simulink model "Main_ekart"  (R2021b)
settings: Solver=FixedStepAuto  StartTime=0.0  StopTime=inf  FixedStep=1/500  RelTol=1e-3  EnableMultiTasking=on
values from neighbouring files (symbols this model uses):
  a = [1 -2.62355180661 2.31468258109 -0.685535977285]    [IMU_filt_100Hz.mat]    (also in IMU_filt_500Hz.mat = [1 -2.92460623545 2.85202781859 -0.92736996835])
  angles = [0 4.9 5 10 15 20 25 30 35 40]    [CreateAllControllers.m]
  b = [0.000699349649901 0.0020980489497 0.0020980489497 0.000699349649901]    [IMU_filt_100Hz.mat]    (also in IMU_filt_500Hz.mat = [6.45184912909e-06 1.93555473873e-05 1.93555473873e-05 6.451)
  D = (DMFx+DMFy)/2    (= 1.2194)    [kart_parameters2.m]
  gear_ratio = 3.2    [kart_parameters2.m]
  L = sys*C    [build_controller_PI.m]    (also in kart_parameters2.m = 1.042)
  newcurrent = [-186.423 -186.283922965 -186.14484593 -186.005768895 -185.866691861 -185.727614826 -185.588537791 -185.449460756 -185.310383721 -185.171306686 -185.032229652 -184.893152617 ... (1000 elements, 1x1000)]    [Torque_map.mat]
  newtorque = [-28.1755 -28.1190925926 -28.0626851852 -28.0062777778 -27.9498703704 -27.893462963 -27.8370555556 -27.7806481481 -27.7242407407 -27.6678333333 -27.6114259259 -27.5550185185 ... (1000 elements, 1x1000)]    [Torque_map.mat]
  percent = [0 0.1001001001 0.2002002002 0.3003003003 0.4004004004 0.500500500501 0.600600600601 0.700700700701 0.800800800801 0.900900900901 1.001001001 1.1011011011 ... (1000 elements, 1x1000)]    [Torque_accel.mat]
  speeds = [0 19.9 20 30 40]    [CreateAllControllers.m]
  table_i = [zeros(1,10) ... (first row only)    [CreateAllControllers.m]
  table_p = [zeros(1, 10) ... (first row only)    [CreateAllControllers.m]
  torque = [0.1025 0.130601101101 0.158702202202 0.186803303303 0.214904404404 0.243005505506 0.271106606607 0.299207707708 0.327308808809 0.35540990991 0.383511011011 0.411612112112 ... (1000 elements, 1x1000)]    [Torque_accel.mat]
libraries: simulink x50, mcp2515lib x46, etargetslib x4, svdutilitieslib x3, cstblocks x2, slpidlib x1
(part 1 of 4)
settings Model: Creator=s393429  LastModifiedBy=maximesabbadini
settings SolverCC: PositivePriorityOrder=on
settings OptimizationCC: EnhancedBackFolding=on  PassReuseOutputArgsThreshold=0  MaxStackSize=64  OptimizeBlockOrder=speed  DifferentSizesBufferReuse=on  OptimizationCustomize=off
settings DebuggingCC: ParameterTunabilityLossMsg=error  UnconnectedInputMsg=none  UnconnectedOutputMsg=none  UnconnectedLineMsg=none
settings HardwareCC: ProdBitPerPointer=32  ProdBitPerSizeT=32  ProdBitPerPtrDiffT=32  ProdLargestAtomicInteger=Long  ProdLargestAtomicFloat=Double  ProdWordSize=32  ProdLongLongMode=on  ProdHWDeviceType=ARM Compatible->ARM Cortex  UseEmbeddedCoderFeatures=off
settings RTWCC: Description=Embedded Coder  SystemTargetFile=ert.tlc  HardwareBoard=Raspberry Pi  TLCOptions="-aInlineSetEventsForThisBaseRateFcn=TLC_FALSE -aSuppressMultiTaskScheduler=TLC_FALSE  -aRateBasedStepFcn=0"  TemplateMakefile=ert_default_tmf  Toolchain=GNU GCC Embedded Linux  BuildConfiguration=Faster Runs  DLArmComputeVersion=20.02.1
settings CodeAppCC: ForceParamTrailComments=on  OperatorAnnotations=on
settings ERTTargetCC: ERTCustomFileBanners=off  SupportContinuousTime=on  SupportNonInlinedSFcns=on  RemoveResetFunc=off  SupportVariableSizeSignals=on  ModelStepFunctionPrototypeControlCompliant=off  ExtMode=on  ExtModeTransport=2  ExtModeStaticAlloc=on  ExtModeMexFile=ext_xcp  ExtModeMexArgs='192.168.8.1' 0 17725  ExtModeIntrfLevel=Level2 - Open  ERTSrcFileBannerTemplate=codertarget_code_template.cgt  ERTHdrFileBannerTemplate=codertarget_code_template.cgt  ERTDataSrcFileTemplate=codertarget_code_template.cgt  ERTDataHdrFileTemplate=codertarget_code_template.cgt

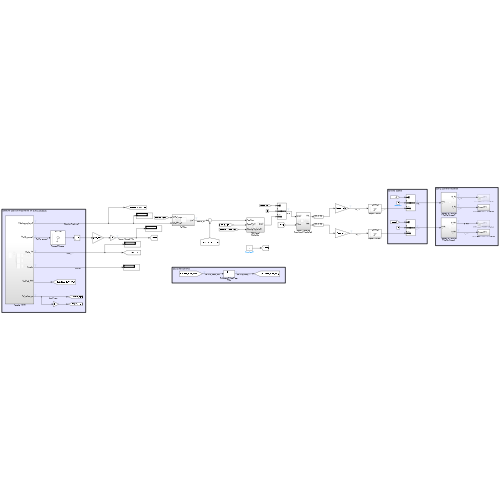
[thumbnail: Simulink's stored preview of the top-level diagram]
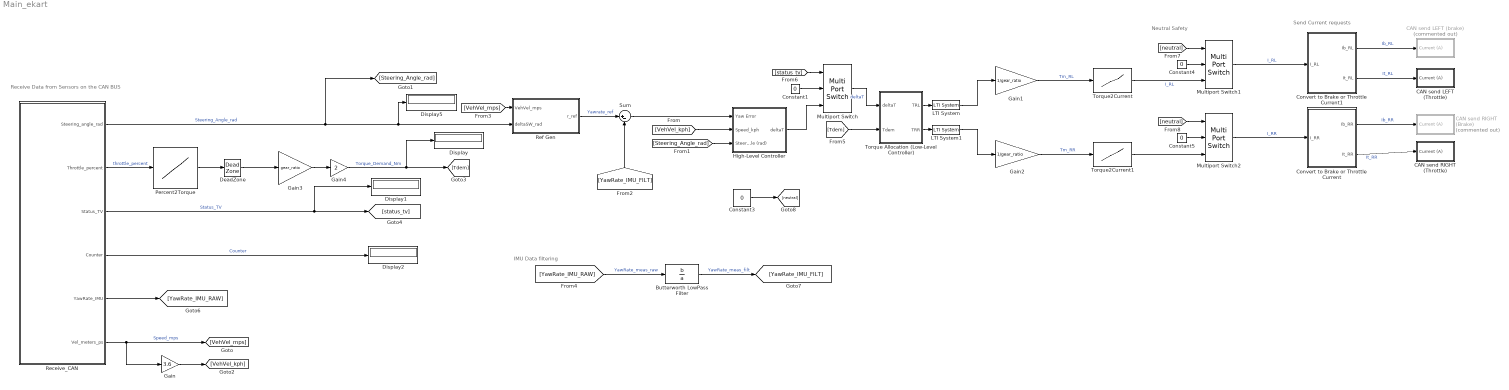
== system Main_ekart ==
  note: Send Current requests
  note: Neutral Safety
  note: IMU Data filtering
  note: Receive Data from Sensors on the CAN BUS
  Butterworth LowPass Filter : DiscreteTransferFcn  Numerator=b  Denominator=a
  CAN send LEFT (Throttle) : Subsystem
  CAN send LEFT (brake) : Subsystem  Commented=on
  CAN send RIGHT (Brake) : Subsystem  Commented=on
  CAN send RIGHT (Throttle) : Subsystem
  Constant1 : Constant  Value=0
  Constant3 : Constant  Value=0
  Constant4 : Constant  Value=0  OutDataTypeStr=int32
  Constant5 : Constant  Value=0  OutDataTypeStr=int32
  Convert to Brake or Throttle Current : Subsystem
  Convert to Brake or Throttle Current1 : Subsystem
  DeadZone : DeadZone  LowerValue=0  UpperValue=1  SaturateOnIntegerOverflow=on
  Display{,1..2,5} (4 alike) : Display
  Gain : Gain  Gain=3.6  OutDataTypeStr=Inherit: Inherit via back propagation
  Gain1 : Gain  Gain=1/gear_ratio
  Gain2 : Gain  Gain=1/gear_ratio
  Gain3 : Gain  Gain=gear_ratio
  Gain4 : Gain  Gain=2
  High-Level Controller : Subsystem
  LTI System : cstblocks/LTI System  sys=tf(5,[1 5])  IC=[]
  LTI System1 : cstblocks/LTI System  sys=tf(5,[1 5])  IC=[]
  Multiport Switch : MultiPortSwitch  DataPortOrder=Zero-based contiguous  Inputs=2  zeroidx=on
  Multiport Switch1 : MultiPortSwitch  DataPortOrder=Zero-based contiguous  Inputs=2  zeroidx=on
  Multiport Switch2 : MultiPortSwitch  DataPortOrder=Zero-based contiguous  Inputs=2  zeroidx=on
  Percent2Torque : Lookup_n-D  NumberOfTableDimensions=1  BreakpointsForDimension1=percent  Table=torque  InternalRulePriority=Speed  RndMeth=Simplest  InputSameDT=on
  Receive_CAN : Subsystem
  Ref Gen : Subsystem
  Sum : Sum  Inputs=|+-
  Torque Allocation (Low-Level Controller) : Subsystem
  Torque2Current : Lookup_n-D  NumberOfTableDimensions=1  BreakpointsForDimension1=newtorque  Table=newcurrent  InternalRulePriority=Speed  RndMeth=Simplest  InputSameDT=on
  Torque2Current1 : Lookup_n-D  NumberOfTableDimensions=1  BreakpointsForDimension1=newtorque  Table=newcurrent  InternalRulePriority=Speed  RndMeth=Simplest  InputSameDT=on
  wires:
  Constant1/1 -> Multiport Switch/2
  High-Level Controller/1(deltaT) -> Multiport Switch/3
  Sum/1 -> High-Level Controller/1(Yaw Error)
  Gain2/1 -> Torque2Current1/1  "Tm_RR"
  Gain1/1 -> Torque2Current/1  "Tm_RL"
  Ref Gen/1(r_ref) -> Sum/1  "Yawrate_ref"
  Torque Allocation (Low-Level Controller)/1(TRL) -> LTI System/1
  Torque Allocation (Low-Level Controller)/2(TRR) -> LTI System1/1
  Multiport Switch/1 -> Torque Allocation (Low-Level Controller)/1(deltaT)  "deltaT"
  [VehVel_kph] -> High-Level Controller/2(Speed_kph)
  [Steering_Angle_rad] -> High-Level Controller/3(Steering Angle (rad))
  [VehVel_mps] -> Ref Gen/1(VehVel_mps)
  Receive_CAN/4(Counter) -> Display2/1  "Counter"
  Percent2Torque/1 -> DeadZone/1
  Torque2Current1/1 -> Multiport Switch2/3
  [neutral] -> Multiport Switch2/1
  [neutral] -> Multiport Switch1/1
  Gain3/1 -> Gain4/1
  Gain4/1 -> [Tdem], Display/1  "Torque_Demand_Nm"
  Receive_CAN/1(Steering_angle_rad) -> [Steering_Angle_rad], Display5/1, Ref Gen/2(deltaSW_rad)  "Steering_Angle_rad"
  LTI System/1 -> Gain1/1
  LTI System1/1 -> Gain2/1
  Receive_CAN/3(Status_TV) -> [status_tv], Display1/1  "Status_TV"
  Convert to Brake or Throttle Current1/1(Ib_RL) -> CAN send LEFT (brake)/1(Current (A))  "Ib_RL"
  [Tdem] -> Torque Allocation (Low-Level Controller)/2(Tdem)
  Receive_CAN/6(Vel_meters_ps) -> Gain/1, [VehVel_mps]  "Speed_mps"
  Gain/1 -> [VehVel_kph]
  Receive_CAN/5(YawRate_IMU) -> [YawRate_IMU_RAW]
  [YawRate_IMU_FILT] -> Sum/2
  [status_tv] -> Multiport Switch/1
  [YawRate_IMU_RAW] -> Butterworth LowPass Filter/1  "YawRate_meas_raw"
  Butterworth LowPass Filter/1 -> [YawRate_IMU_FILT]  "YawRate_meas_filt"
  DeadZone/1 -> Gain3/1
  Convert to Brake or Throttle Current1/2(It_RL) -> CAN send LEFT (Throttle)/1(Current (A))  "It_RL"
  Constant3/1 -> [neutral]
  Convert to Brake or Throttle Current/2(It_RR) -> CAN send RIGHT (Throttle)/1(Current (A))  "It_RR"
  Receive_CAN/2(Throttle_percent) -> Percent2Torque/1  "throttle_percent"
  Constant5/1 -> Multiport Switch2/2
  Constant4/1 -> Multiport Switch1/2
  Torque2Current/1 -> Multiport Switch1/3  "I_RL"
  Multiport Switch2/1 -> Convert to Brake or Throttle Current/1(I_RR)  "I_RR"
  Convert to Brake or Throttle Current/1(Ib_RR) -> CAN send RIGHT (Brake)/1(Current (A))  "Ib_RR"
  Multiport Switch1/1 -> Convert to Brake or Throttle Current1/1(I_RL)  "I_RL"

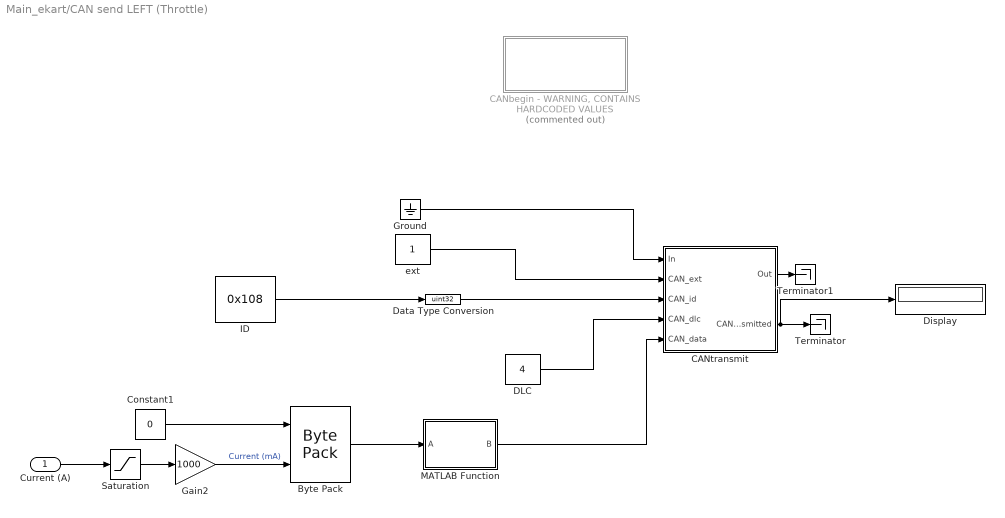
== system Main_ekart/CAN send LEFT (Throttle) ==
  Current (A) : Inport  OutDataTypeStr=int32  PortDimensions=1
  Byte Pack : etargetslib/Byte Pack  datatypes={'int32','int32'}  byteAlign=1
  "CANbegin - WARNING, CONTAINS HARDCODED VALUES" : Subsystem  Commented=on  TreatAsAtomicUnit=on  mask{TargetHardware=Raspberry Pi, Oscillator=10, CANSpeed=500, CSpin=10}
      mask prompts: TargetHardware "Target Hardware"; Oscillator "Oscillator frequency(MHz)"; CANSpeed "CAN speed(kHz)"; CSpin "Chip Select Pin"
      mask init:
      | % Get this mask's handle
      | maskObj = Simulink.Mask.get(gcb);
      | 
      | % Get the selected value from mask parameter's option
      | str_TargetHard = char(maskObj.Parameters(1).TypeOptions(TargetHardware));
      | str_Osc = char(maskObj.Parameters(2).TypeOptions(Oscillator));
      | str_CANSpeed = char(maskObj.Parameters(3).TypeOptions(CANSpeed));
      | 
      | % Set Icon
      | str1 = sprintf('%s(Model)',str_TargetHard);
      | str2 = sprintf('Oscillator: %s(MHz)',str_Osc);
      | str3 = sprintf('CAN Bus Speed: %s(kHz)',str_CANSpeed);
      | str4 = sprintf('Chip Select pin: %d',CSpin);
      | 
      | % Set the values of Variant Subsystem
      | switch str_TargetHard
      |     case 'Arduino'
      |         str = [str1,'\n',str2,'\n',str3,'\n',str4];
      |         evalin('base',sprintf('CSpin = %d;',CSpin));        
      |         evalin('base','Hardware = 1;');
      |     case 'Raspberry Pi'
      |         str = [str1,'\n',str2,'\n',str3];
      |         evalin('base',sprintf('clear CSpin',CSpin));           
      |         evalin('base','Hardware = 2;');     
      | end  
      | 
      | % Get the CAN Configuration register's value from mask parameter's option
      | if str_Osc == '8' %[MHz]
      |     switch str_CANSpeed
      |         case '1000'
      |             BPR = 0; PHSEG1 = 0; PRSEG = 0; PHSEG2 = 0;
      |         case '500'
      |             BPR = 0; PHSEG1 = 2; PRSEG = 0; PHSEG2 = 2;
      |         case '250'
      |             BPR = 0; PHSEG1 = 6; PRSEG = 0; PHSEG2 = 6;
      |         case '125'
      |             BPR = 1; PHSEG1 = 6; PRSEG = 1; PHSEG2 = 5;
      |         case '100'
      |             BPR = 1; PHSEG1 = 7; PRSEG = 2; PHSEG2 = 7;
      |         case '83.3'
      |             BPR = 1; PHSEG1 = 7; PRSEG = 6; PHSEG2 = 7;
      |         case '62.5'
      |             BPR = 3; PHSEG1 = 6; PRSEG = 0; PHSEG2 = 6;
      |         case '50'
      |             BPR = 3; PHSEG1 = 7; PRSEG = 2; PHSEG2 = 7;
      |         case '33.3'
      |             BPR = 4; PHSEG1 = 7; PRSEG = 6; PHSEG2 = 7;
      |     end            
      | elseif str_Osc == '16' %[MHz]
      |     switch str_CANSpeed  
      |         case '1000'
      |             BPR = 0; PHSEG1 = 2; PRSEG = 0; PHSEG2 = 2;
      |         case '500'
      |             BPR = 0; PHSEG1 = 6; PRSEG = 0; PHSEG2 = 6;
      |         case '250'
      |             BPR = 1; PHSEG1 = 6; PRSEG = 1; PHSEG2 = 5;        
      |         case '125'
      |             BPR = 3; PHSEG1 = 6; PRSEG = 0; PHSEG2 = 6;
      |         case '100'
      |             BPR = 3; PHSEG1 = 7; PRSEG = 2; PHSEG2 = 7;
      |         case '83.3'
      |             BPR = 3; PHSEG1 = 7; PRSEG = 6; PHSEG2 = 7;
      |         case '62.5'
      |             BPR = 7; PHSEG1 = 6; PRSEG = 0; PHSEG2 = 6;
      |         case '50'
      |             BPR = 7; PHSEG1 = 7; PRSEG = 2; PHSEG2 = 7;
      |         case '33.3'
      |             BPR = 9; PHSEG1 = 7; PRSEG = 6; PHSEG2 = 7;        
      |     end
      |     
      | elseif str_Osc == '10' %[MHz]
      |     switch str_CANSpeed  
      |         case '1000'
      |             BPR = 0; PHSEG1 = 2; PRSEG = 0; PHSEG2 = 2;
      |         case '500'
      |             BPR = 0; PHSEG1 = 5; PRSEG = 0; PHSEG2 = 4;
      |         case '250'
      |             BPR = 1; PHSEG1 = 6; PRSEG = 1; PHSEG2 = 5;        
      |         case '125'
      |             BPR = 3; PHSEG1 = 6; PRSEG = 0; PHSEG2 = 6;
      |         case '100'
      |             BPR = 3; PHSEG1 = 7; PRSEG = 2; PHSEG2 = 7;
      |         case '83.3'
      |             BPR = 3; PHSEG1 = 7; PRSEG = 6; PHSEG2 = 7;
      |         case '62.5'
      |             BPR = 7; PHSEG1 = 6; PRSEG = 0; PHSEG2 = 6;
      |         case '50'
      |             BPR = 7; PHSEG1 = 7; PRSEG = 2; PHSEG2 = 7;
      |         case '33.3'
      |             BPR = 9; PHSEG1 = 7; PRSEG = 6; PHSEG2 = 7;        
      |     end    
      |     
      |     
      | end
      | % % Set the CAN Configuration register's value
      | % address2A = BPR;          % bit7-6 :SJW, bit5-0: BPR
      | % address29 = 192 ...       % bit7: BTLMODE = 1, bit6:SAM = 1
      | %             + 8*PHSEG1 ...% bit5-3: PHSEG1
      | %             +PRSEG;       % bit2-0: PRSEG
      | % address28 = 128 ...       % bit7: SOF = 1, bit6:WAKFIL = 0
      | %             + PHSEG2;     % bit5-3: 0, bit2-0: PHSEG2
      |         
      | % force parameters... 
      | % %1M CAN
      | % address2A=hex2dec('40')
      | % address29=hex2dec('80')
      | % address28=hex2dec('1')
      | 
      | %500k CAN
      | address2A=hex2dec('0')
      | address29=hex2dec('A0')
      | address28=hex2dec('02')
      | 
      | % %500k CAN from Arduino library spreadsheet - doesn't work
      | % address2A=hex2dec('41')
      | % address29=hex2dec('D9')
      | % address28=hex2dec('82')
      settings: RTWSystemCode=Nonreusable function
      mask TypeOptions TargetHardware: Arduino | Raspberry Pi
      mask Callback TargetHardware:
      | if(strcmp(get_param(gcb,'TargetHardware'),'Arduino'))
      |     set_param(gcb,'MaskVisibilities',{'on','on','on','on'})
      | else
      |     set_param(gcb,'MaskVisibilities',{'on','on','on','off'})
      | end
      mask TypeOptions Oscillator: 8 | 16 | 10
      mask TypeOptions CANSpeed: 1000 | 500 | 250 | 125 | 100 | 83.3 | 62.5 | 50 | 33.3
      mask DialogControl DescGroupVar Prompt: Description
      mask DialogControl DescTextVar Prompt: Forced parameters for 10MHz oscillator, 500k CAN This block must be executed only once when beginning CAN communication because MCP2515’s register needs to be configured. And the frequency of oscillator for MCP2515 is also needed because it effects to the setting parameters of MCP2515's register.
      mask Display: disp(str)
  CANtransmit : Subsystem  TreatAsAtomicUnit=on
      mask DialogControl DescGroupVar Prompt: Description
      mask DialogControl DescTextVar Prompt: CANtransmit inputs CAN data by converting MCP2515 TX buffer register’s values. In/Out ports are no use because they are used for controlling the execution order. CAN_Transmitted outputs 1(Success) or 2(Fail).
  Constant1 : Constant  Value=0  OutDataTypeStr=int32
  DLC : Constant  Value=4  OutDataTypeStr=uint8
  Data Type Conversion : DataTypeConversion  OutDataTypeStr=uint32
  Display : Display
  Gain2 : Gain  Gain=1000  OutDataTypeStr=int32
  Ground : Ground
  ID : Constant  Value=0x108  OutDataTypeStr=uint32
  MATLAB Function : MATLAB Function  TreatAsAtomicUnit=on
  Saturation : Saturate  UpperLimit=180  LowerLimit=0  OutDataTypeStr=int32
  Terminator : Terminator
  Terminator1 : Terminator
  ext : Constant  OutDataTypeStr=uint8
  wires:
  Byte Pack/1 -> MATLAB Function/1(A)
  Ground/1 -> CANtransmit/1(In)
  ext/1 -> CANtransmit/2(CAN_ext)
  DLC/1 -> CANtransmit/4(CAN_dlc)
  ID/1 -> Data Type Conversion/1
  CANtransmit/1(Out) -> Terminator1/1
  CANtransmit/2(CAN_Transmitted) -> Display/1, Terminator/1
  Constant1/1 -> Byte Pack/1
  Current (A)/1 -> Saturation/1
  MATLAB Function/1(B) -> CANtransmit/5(CAN_data)
  Saturation/1 -> Gain2/1
  Gain2/1 -> Byte Pack/2  "Current (mA)"
  Data Type Conversion/1 -> CANtransmit/3(CAN_id)

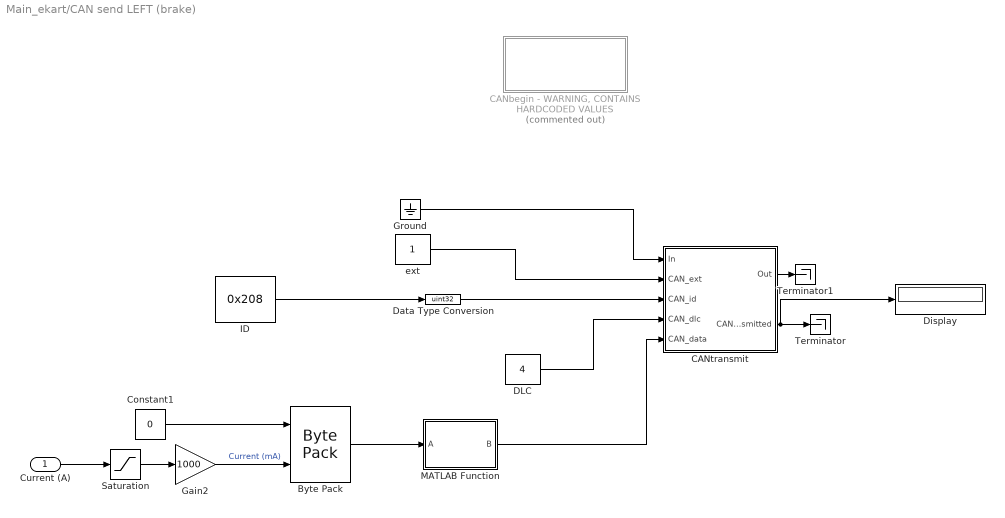
== system Main_ekart/CAN send LEFT (brake) ==
  Current (A) : Inport  OutDataTypeStr=int32  PortDimensions=1
  Byte Pack : etargetslib/Byte Pack  datatypes={'int32','int32'}  byteAlign=1
  "CANbegin - WARNING, CONTAINS HARDCODED VALUES" : Subsystem  Commented=on  TreatAsAtomicUnit=on  mask{TargetHardware=Raspberry Pi, Oscillator=10, CANSpeed=500, CSpin=10}
      mask prompts: TargetHardware "Target Hardware"; Oscillator "Oscillator frequency(MHz)"; CANSpeed "CAN speed(kHz)"; CSpin "Chip Select Pin"
      mask init: same as Main_ekart/CAN send LEFT (Throttle)/CANbegin - WARNING, CONTAINS HARDCODED VALUES
      settings: RTWSystemCode=Nonreusable function
      mask TypeOptions TargetHardware: Arduino | Raspberry Pi
      mask Callback TargetHardware:
      | if(strcmp(get_param(gcb,'TargetHardware'),'Arduino'))
      |     set_param(gcb,'MaskVisibilities',{'on','on','on','on'})
      | else
      |     set_param(gcb,'MaskVisibilities',{'on','on','on','off'})
      | end
      mask TypeOptions Oscillator: 8 | 16 | 10
      mask TypeOptions CANSpeed: 1000 | 500 | 250 | 125 | 100 | 83.3 | 62.5 | 50 | 33.3
      mask DialogControl DescGroupVar Prompt: Description
      mask DialogControl DescTextVar Prompt: Forced parameters for 10MHz oscillator, 500k CAN This block must be executed only once when beginning CAN communication because MCP2515’s register needs to be configured. And the frequency of oscillator for MCP2515 is also needed because it effects to the setting parameters of MCP2515's register.
      mask Display: disp(str)
  CANtransmit : Subsystem  TreatAsAtomicUnit=on
      mask DialogControl DescGroupVar Prompt: Description
      mask DialogControl DescTextVar Prompt: CANtransmit inputs CAN data by converting MCP2515 TX buffer register’s values. In/Out ports are no use because they are used for controlling the execution order. CAN_Transmitted outputs 1(Success) or 2(Fail).
  Constant1 : Constant  Value=0  OutDataTypeStr=int32
  DLC : Constant  Value=4  OutDataTypeStr=uint8
  Data Type Conversion : DataTypeConversion  OutDataTypeStr=uint32
  Display : Display
  Gain2 : Gain  Gain=1000  OutDataTypeStr=int32
  Ground : Ground
  ID : Constant  Value=0x208  OutDataTypeStr=uint32
  MATLAB Function : MATLAB Function  TreatAsAtomicUnit=on
  Saturation : Saturate  UpperLimit=180  LowerLimit=0  OutDataTypeStr=int32
  Terminator : Terminator
  Terminator1 : Terminator
  ext : Constant  OutDataTypeStr=uint8
  wires:
  Data Type Conversion/1 -> CANtransmit/3(CAN_id)
  Gain2/1 -> Byte Pack/2  "Current (mA)"
  Saturation/1 -> Gain2/1
  MATLAB Function/1(B) -> CANtransmit/5(CAN_data)
  Current (A)/1 -> Saturation/1
  Constant1/1 -> Byte Pack/1
  CANtransmit/2(CAN_Transmitted) -> Terminator/1, Display/1
  CANtransmit/1(Out) -> Terminator1/1
  ID/1 -> Data Type Conversion/1
  DLC/1 -> CANtransmit/4(CAN_dlc)
  ext/1 -> CANtransmit/2(CAN_ext)
  Ground/1 -> CANtransmit/1(In)
  Byte Pack/1 -> MATLAB Function/1(A)

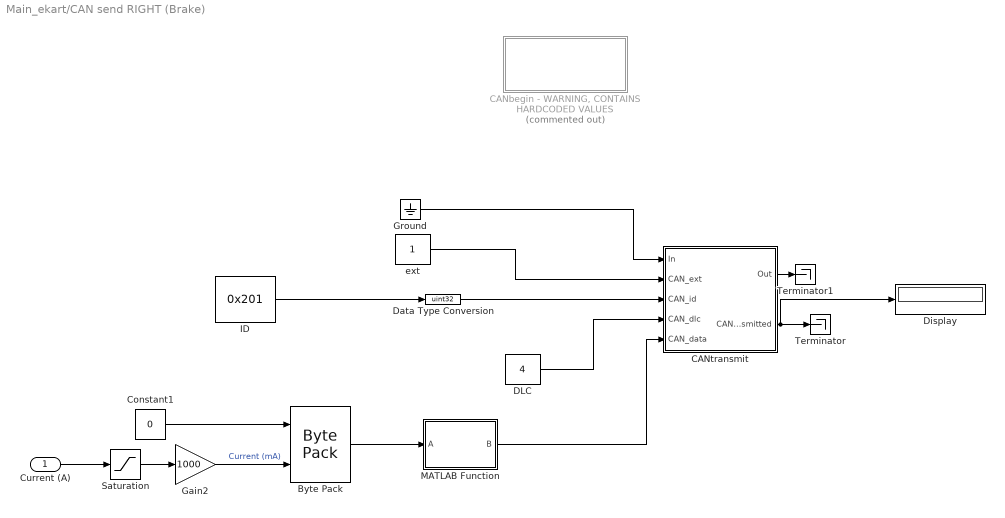
== system Main_ekart/CAN send RIGHT (Brake) ==
  Current (A) : Inport  OutDataTypeStr=int32  PortDimensions=1
  Byte Pack : etargetslib/Byte Pack  datatypes={'int32','int32'}  byteAlign=1
  "CANbegin - WARNING, CONTAINS HARDCODED VALUES" : Subsystem  Commented=on  TreatAsAtomicUnit=on  mask{TargetHardware=Raspberry Pi, Oscillator=10, CANSpeed=500, CSpin=10}
      mask prompts: TargetHardware "Target Hardware"; Oscillator "Oscillator frequency(MHz)"; CANSpeed "CAN speed(kHz)"; CSpin "Chip Select Pin"
      mask init: same as Main_ekart/CAN send LEFT (Throttle)/CANbegin - WARNING, CONTAINS HARDCODED VALUES
      settings: RTWSystemCode=Nonreusable function
      mask TypeOptions TargetHardware: Arduino | Raspberry Pi
      mask Callback TargetHardware:
      | if(strcmp(get_param(gcb,'TargetHardware'),'Arduino'))
      |     set_param(gcb,'MaskVisibilities',{'on','on','on','on'})
      | else
      |     set_param(gcb,'MaskVisibilities',{'on','on','on','off'})
      | end
      mask TypeOptions Oscillator: 8 | 16 | 10
      mask TypeOptions CANSpeed: 1000 | 500 | 250 | 125 | 100 | 83.3 | 62.5 | 50 | 33.3
      mask DialogControl DescGroupVar Prompt: Description
      mask DialogControl DescTextVar Prompt: Forced parameters for 10MHz oscillator, 500k CAN This block must be executed only once when beginning CAN communication because MCP2515’s register needs to be configured. And the frequency of oscillator for MCP2515 is also needed because it effects to the setting parameters of MCP2515's register.
      mask Display: disp(str)
  CANtransmit : Subsystem  TreatAsAtomicUnit=on
      mask DialogControl DescGroupVar Prompt: Description
      mask DialogControl DescTextVar Prompt: CANtransmit inputs CAN data by converting MCP2515 TX buffer register’s values. In/Out ports are no use because they are used for controlling the execution order. CAN_Transmitted outputs 1(Success) or 2(Fail).
  Constant1 : Constant  Value=0  OutDataTypeStr=int32
  DLC : Constant  Value=4  OutDataTypeStr=uint8
  Data Type Conversion : DataTypeConversion  OutDataTypeStr=uint32
  Display : Display
  Gain2 : Gain  Gain=1000  OutDataTypeStr=int32
  Ground : Ground
  ID : Constant  Value=0x201  OutDataTypeStr=uint32
  MATLAB Function : MATLAB Function  TreatAsAtomicUnit=on
  Saturation : Saturate  UpperLimit=180  LowerLimit=0  OutDataTypeStr=int32
  Terminator : Terminator
  Terminator1 : Terminator
  ext : Constant  OutDataTypeStr=uint8
  wires:
  Byte Pack/1 -> MATLAB Function/1(A)
  Ground/1 -> CANtransmit/1(In)
  ext/1 -> CANtransmit/2(CAN_ext)
  DLC/1 -> CANtransmit/4(CAN_dlc)
  ID/1 -> Data Type Conversion/1
  CANtransmit/1(Out) -> Terminator1/1
  CANtransmit/2(CAN_Transmitted) -> Display/1, Terminator/1
  Constant1/1 -> Byte Pack/1
  Current (A)/1 -> Saturation/1
  MATLAB Function/1(B) -> CANtransmit/5(CAN_data)
  Saturation/1 -> Gain2/1
  Gain2/1 -> Byte Pack/2  "Current (mA)"
  Data Type Conversion/1 -> CANtransmit/3(CAN_id)

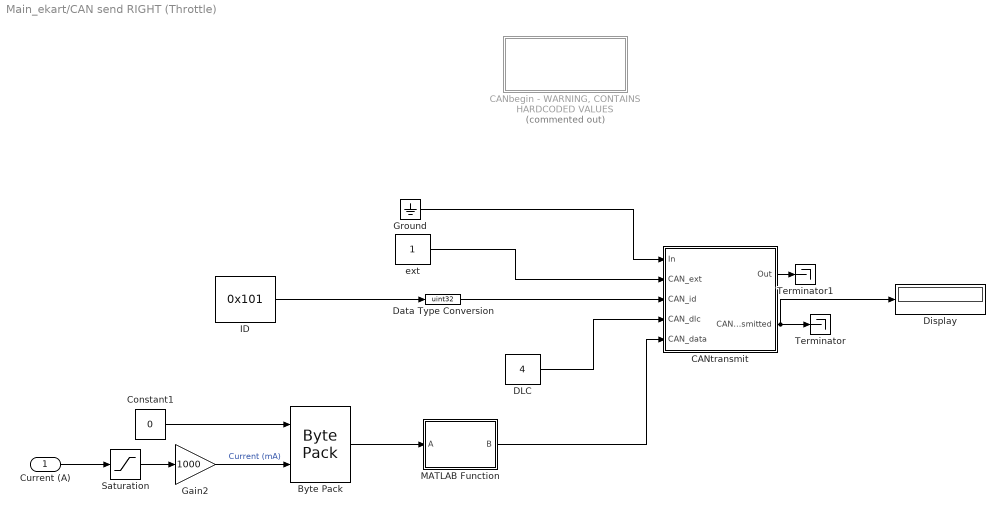
== system Main_ekart/CAN send RIGHT (Throttle) ==
  Current (A) : Inport  OutDataTypeStr=int32  PortDimensions=1
  Byte Pack : etargetslib/Byte Pack  datatypes={'int32','int32'}  byteAlign=1
  "CANbegin - WARNING, CONTAINS HARDCODED VALUES" : Subsystem  Commented=on  TreatAsAtomicUnit=on  mask{TargetHardware=Raspberry Pi, Oscillator=10, CANSpeed=500, CSpin=10}
      mask prompts: TargetHardware "Target Hardware"; Oscillator "Oscillator frequency(MHz)"; CANSpeed "CAN speed(kHz)"; CSpin "Chip Select Pin"
      mask init: same as Main_ekart/CAN send LEFT (Throttle)/CANbegin - WARNING, CONTAINS HARDCODED VALUES
      settings: RTWSystemCode=Nonreusable function
      mask TypeOptions TargetHardware: Arduino | Raspberry Pi
      mask Callback TargetHardware:
      | if(strcmp(get_param(gcb,'TargetHardware'),'Arduino'))
      |     set_param(gcb,'MaskVisibilities',{'on','on','on','on'})
      | else
      |     set_param(gcb,'MaskVisibilities',{'on','on','on','off'})
      | end
      mask TypeOptions Oscillator: 8 | 16 | 10
      mask TypeOptions CANSpeed: 1000 | 500 | 250 | 125 | 100 | 83.3 | 62.5 | 50 | 33.3
      mask DialogControl DescGroupVar Prompt: Description
      mask DialogControl DescTextVar Prompt: Forced parameters for 10MHz oscillator, 500k CAN This block must be executed only once when beginning CAN communication because MCP2515’s register needs to be configured. And the frequency of oscillator for MCP2515 is also needed because it effects to the setting parameters of MCP2515's register.
      mask Display: disp(str)
  CANtransmit : Subsystem  TreatAsAtomicUnit=on
      mask DialogControl DescGroupVar Prompt: Description
      mask DialogControl DescTextVar Prompt: CANtransmit inputs CAN data by converting MCP2515 TX buffer register’s values. In/Out ports are no use because they are used for controlling the execution order. CAN_Transmitted outputs 1(Success) or 2(Fail).
  Constant1 : Constant  Value=0  OutDataTypeStr=int32
  DLC : Constant  Value=4  OutDataTypeStr=uint8
  Data Type Conversion : DataTypeConversion  OutDataTypeStr=uint32
  Display : Display
  Gain2 : Gain  Gain=1000  OutDataTypeStr=int32
  Ground : Ground
  ID : Constant  Value=0x101  OutDataTypeStr=uint32
  MATLAB Function : MATLAB Function  TreatAsAtomicUnit=on
  Saturation : Saturate  UpperLimit=180  LowerLimit=0  OutDataTypeStr=int32
  Terminator : Terminator
  Terminator1 : Terminator
  ext : Constant  OutDataTypeStr=uint8
  wires:
  Data Type Conversion/1 -> CANtransmit/3(CAN_id)
  Gain2/1 -> Byte Pack/2  "Current (mA)"
  Saturation/1 -> Gain2/1
  MATLAB Function/1(B) -> CANtransmit/5(CAN_data)
  Current (A)/1 -> Saturation/1
  Constant1/1 -> Byte Pack/1
  CANtransmit/2(CAN_Transmitted) -> Terminator/1, Display/1
  CANtransmit/1(Out) -> Terminator1/1
  ID/1 -> Data Type Conversion/1
  DLC/1 -> CANtransmit/4(CAN_dlc)
  ext/1 -> CANtransmit/2(CAN_ext)
  Ground/1 -> CANtransmit/1(In)
  Byte Pack/1 -> MATLAB Function/1(A)

== system Main_ekart/Convert to Brake or Throttle Current ==
  I_RR : Inport
  Compare To Constant1 : simulink/Logic and Bit Operations/Compare To Constant  relop=<=  const=0  OutDataTypeStr=boolean
  Data Type Conversion5 : DataTypeConversion  OutDataTypeStr=int32
  Data Type Conversion6 : DataTypeConversion  OutDataTypeStr=int32
  MATLAB Function1 : MATLAB Function  TreatAsAtomicUnit=on
  Ib_RR : Outport
  It_RR : Outport  Port=2
  wires:
  Data Type Conversion5/1 -> Ib_RR/1  "Ib_RR"
  Data Type Conversion6/1 -> It_RR/1  "It_RR"
  Compare To Constant1/1 -> MATLAB Function1/1(sign_current)
  MATLAB Function1/1(brake_current) -> Data Type Conversion5/1
  MATLAB Function1/2(throttle_current) -> Data Type Conversion6/1
  I_RR/1 -> MATLAB Function1/2(current), Compare To Constant1/1

== system Main_ekart/Convert to Brake or Throttle Current1 ==
  I_RL : Inport
  Compare To Constant1 : simulink/Logic and Bit Operations/Compare To Constant  relop=<=  const=0  OutDataTypeStr=boolean
  Data Type Conversion5 : DataTypeConversion  OutDataTypeStr=int32
  Data Type Conversion6 : DataTypeConversion  OutDataTypeStr=int32
  MATLAB Function1 : MATLAB Function  TreatAsAtomicUnit=on
  Ib_RL : Outport
  It_RL : Outport  Port=2
  wires:
  Data Type Conversion5/1 -> Ib_RL/1  "Ib_RR"
  Data Type Conversion6/1 -> It_RL/1  "It_RR"
  Compare To Constant1/1 -> MATLAB Function1/1(sign_current)
  MATLAB Function1/1(brake_current) -> Data Type Conversion5/1
  MATLAB Function1/2(throttle_current) -> Data Type Conversion6/1
  I_RL/1 -> MATLAB Function1/2(current), Compare To Constant1/1

== system Main_ekart/High-Level Controller ==
  Yaw Error : Inport
  Speed_kph : Inport  Port=2
  Steering Angle (rad) : Inport  Port=3
  Abs : Abs
  Constant : Constant  Value=0
  Constant1 : Constant  Value=0
  Gain : Gain  Gain=180/pi
  Integral Gain : Lookup_n-D  BreakpointsForDimension1=speeds  BreakpointsForDimension2=angles  BreakpointsForDimension3=[5, 7]  Table=table_i  InternalRulePriority=Speed  RndMeth=Simplest  InputSameDT=on
      settings: InputPortMap=u0,u1
  PID Controller : slpidlib/PID Controller  Controller=PID  Form=Parallel  TimeDomain=Continuous-time  UseExternalTs=off  SampleTime=-1  IntegratorMethod=Forward Euler  FilterMethod=Forward Euler  ControllerParametersSource=external  P=1  I=1  D=0  UseFilter=on  N=100  TunerSelectOption=Transfer Function Based (PID Tuner App)  InitialConditionSource=internal  InitialConditionForIntegrator=0  InitialConditionForFilter=0  DifferentiatorICPrevScaledInput=0  ExternalReset=none  TrackingMode=off  Kt=1  LimitOutput=off  SatLimitsSource=internal  UpperSaturationLimit=inf  LowerSaturationLimit=-inf  LinearizeAsGain=on  AntiWindupMode=none  Kb=1  POutMin=[]  POutMax=[]  IOutMin=[]  IOutMax=[]  DOutMin=[]  DOutMax=[]  NOutMin=[]  NOutMax=[]  SumOutMin=[]  SumOutMax=[]  SaturationOutMin=[]  SaturationOutMax=[]  PParamMin=[]  PParamMax=[]  IParamMin=[]  IParamMax=[]  DParamMin=[]  DParamMax=[]  NParamMin=[]  NParamMax=[]  KbParamMin=[]  KbParamMax=[]  KtParamMin=[]  KtParamMax=[]  KbOutMin=[]  KbOutMax=[]  KtOutMin=[]  KtOutMax=[]  IntegratorOutMin=[]  IntegratorOutMax=[]  FilterOutMin=[]  FilterOutMax=[]  SumI1OutMin=[]  SumI1OutMax=[]  SumI2OutMin=[]  SumI2OutMax=[]  SumI3OutMin=[]  SumI3OutMax=[]  SumI4OutMin=[]  SumI4OutMax=[]  SumDOutMin=[]  SumDOutMax=[]  DifferentiatorOutMin=[]  DifferentiatorOutMax=[]  FilterDiffOutCoefMin=[]  FilterDiffOutCoefMax=[]  ReciprocalOutMin=[]  ReciprocalOutMax=[]  SumDenOutMin=[]  SumDenOutMax=[]  SumNumOutMin=[]  SumNumOutMax=[]  DivideOutMin=[]  DivideOutMax=[]  UdiffTsProdOutMin=[]  UdiffTsProdOutMax=[]  NTsProdOutMin=[]  NTsProdOutMax=[]  UintegralTsProdOutMin=[]  UintegralTsProdOutMax=[]  UngainTsProdOutMin=[]  UngainTsProdOutMax=[]  IntegratorContinuousStateAttributes=''  IntegratorStateMustResolveToSignalObject=off  IntegratorRTWStateStorageClass=Auto  FilterContinuousStateAttributes=''  FilterStateMustResolveToSignalObject=off  FilterRTWStateStorageClass=Auto  ParallelPVariant=ExternalParameters  IdealPVariant=Disabled  IVariant=ExternalParameters  DVariant=ExternalParameters  IntegratorVariant=Continuous  SatVariant=Disabled  AWVariant=Passthrough  PCopyVariant=Disabled  TRVariant=Disabled  FdbkBlocksVariant=Forward  IdealPFdbkVariant=Disabled  SatFdbkVariant=Disabled  DerivativeFilterVariant=ContFilter  NVariant=ExternalParameters  NCopyVariant=Disabled  FilterICVariant=InternalICsFilter  IntegratorICVariant=InternalICs  ExternalResetVariant=Disabled  TRSumVariant=Passthrough  SumFdbkVariant=Disabled  SumVariant=Sum_PID  TsampFilterVariant=InternalTs  TsampNgainVariant=Passthrough  TsampIntegralVariant=Passthrough  ExternalSaturationOutDataTypeStr=Inherit: Same as second input
  Proportional Gain : Lookup_n-D  BreakpointsForDimension1=speeds  BreakpointsForDimension2=angles  BreakpointsForDimension3=[5, 7]  Table=table_p  InternalRulePriority=Speed  RndMeth=Simplest  InputSameDT=on
      settings: InputPortMap=u0,u1
  deltaT : Outport
  wires:
  Yaw Error/1 -> PID Controller/1
  Speed_kph/1 -> Integral Gain/1, Proportional Gain/1
  Steering Angle (rad)/1 -> Gain/1
  Proportional Gain/1 -> PID Controller/2
  Constant/1 -> PID Controller/4
  Constant1/1 -> PID Controller/5
  Integral Gain/1 -> PID Controller/3
  PID Controller/1 -> deltaT/1
  Gain/1 -> Abs/1
  Abs/1 -> Proportional Gain/2, Integral Gain/2

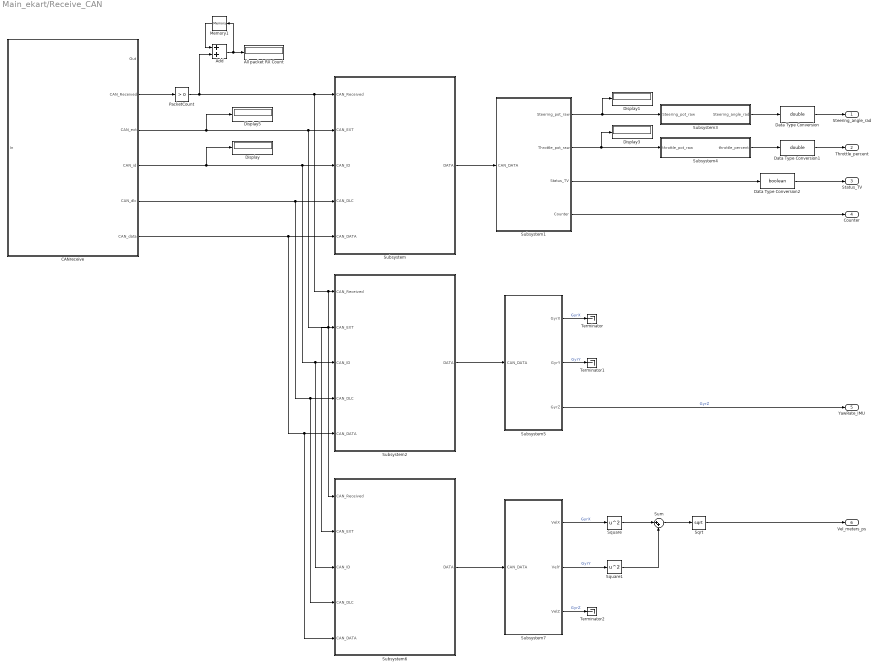
== system Main_ekart/Receive_CAN ==
  Add : Sum  OutDataTypeStr=uint32
  All packet RX Count : Display
  CANreceive : Subsystem  TreatAsAtomicUnit=on
      mask DialogControl DescGroupVar Prompt: Description
      mask DialogControl DescTextVar Prompt: CANreceive outputs CAN data by converting MCP2515 RX buffer register’s values. In/Out ports are no use because they are used for controlling the execution order. CAN_Received outputs 1(CAN received) or -1( No message).
  Data Type Conversion : DataTypeConversion  OutDataTypeStr=double
  Data Type Conversion1 : DataTypeConversion  OutDataTypeStr=double
  Data Type Conversion2 : DataTypeConversion  OutDataTypeStr=boolean
  Display{,1,3,5} (4 alike) : Display
      Display settings: Format=hex (Stored Integer)
  Memory1 : Memory  InitialCondition=[0]
  "PacketCount " : simulink/Logic and Bit Operations/Compare To Constant  relop=>  const=0  OutDataTypeStr=uint8
  Sqrt : Sqrt  SaturateOnIntegerOverflow=on
  Square : Math  Operator=square  SaturateOnIntegerOverflow=on
  Square1 : Math  Operator=square  SaturateOnIntegerOverflow=on
  Subsystem : Subsystem  mask{ID=0x123, DLC=6, EXT=1}
      mask prompts: ID "Message ID"; DLC "Message DLC"; EXT "Type of ID (1 is extended, 0 is standard)"
      mask DialogControl DescGroupVar Prompt: Filter CAN Data
      mask DialogControl DescTextVar Prompt: Give the ID and DLC of the CAN Message you want to get the data from
  Subsystem1 : Subsystem
  Subsystem2 : Subsystem  mask{ID=0x32, DLC=6, EXT=1}
      mask prompts: ID "Message ID"; DLC "Message DLC"; EXT "Type of ID (1 is extended, 0 is standard)"
      mask DialogControl DescGroupVar Prompt: Filter CAN Data
      mask DialogControl DescTextVar Prompt: Give the ID and DLC of the CAN Message you want to get the data from
  Subsystem3 : Subsystem
  Subsystem4 : Subsystem
  Subsystem5 : Subsystem
  Subsystem6 : Subsystem  mask{ID=0x76, DLC=6, EXT=1}
      mask prompts: ID "Message ID"; DLC "Message DLC"; EXT "Type of ID (1 is extended, 0 is standard)"
      mask DialogControl DescGroupVar Prompt: Filter CAN Data
      mask DialogControl DescTextVar Prompt: Give the ID and DLC of the CAN Message you want to get the data from
  Subsystem7 : Subsystem
  Sum : Sum  Inputs=|++
  Terminator : Terminator
  Terminator1 : Terminator
  Terminator2 : Terminator
  Steering_angle_rad : Outport
  Throttle_percent : Outport  Port=2
  Status_TV : Outport  Port=3
  Counter : Outport  Port=4
  YawRate_IMU : Outport  Port=5
  Vel_meters_ps : Outport  Port=6
  wires:
  Subsystem1/1(Steering_pot_raw) -> Subsystem3/1(Steering_pot_raw), Display1/1
  Subsystem1/4(Counter) -> Counter/1
  Subsystem3/1(Steering_angle_rad) -> Data Type Conversion/1
  Subsystem1/2(Throttle_pot_raw) -> Subsystem4/1(throttle_pot_raw), Display3/1
  Subsystem1/3(Status_TV) -> Data Type Conversion2/1
  Memory1/1 -> Add/1
  CANreceive/4(CAN_id) -> Display/1, Subsystem/3(CAN_ID), Subsystem2/3(CAN_ID), Subsystem6/3(CAN_ID)
  Subsystem/1(DATA) -> Subsystem1/1(CAN_DATA)
  Subsystem4/1(throttle_percent) -> Data Type Conversion1/1
  CANreceive/3(CAN_ext) -> Display5/1, Subsystem/2(CAN_EXT), Subsystem6/2(CAN_EXT), Subsystem2/2(CAN_EXT)
  CANreceive/6(CAN_data) -> Subsystem/5(CAN_DATA), Subsystem6/5(CAN_DATA), Subsystem2/5(CAN_DATA)
  CANreceive/5(CAN_dlc) -> Subsystem2/4(CAN_DLC), Subsystem6/4(CAN_DLC), Subsystem/4(CAN_DLC)
  CANreceive/2(CAN_Received) -> "PacketCount "/1
  "PacketCount "/1 -> Add/2, Subsystem/1(CAN_Received), Subsystem6/1(CAN_Received), Subsystem2/1(CAN_Received)
  Add/1 -> All packet RX Count/1, Memory1/1
  Data Type Conversion/1 -> Steering_angle_rad/1
  Data Type Conversion1/1 -> Throttle_percent/1
  Data Type Conversion2/1 -> Status_TV/1
  Subsystem2/1(DATA) -> Subsystem5/1(CAN_DATA)
  Subsystem5/1(GyrX) -> Terminator/1  "GyrX"
  Subsystem5/2(GyrY) -> Terminator1/1  "GyrY"
  Subsystem5/3(GyrZ) -> YawRate_IMU/1  "GyrZ"
  Subsystem6/1(DATA) -> Subsystem7/1(CAN_DATA)
  Subsystem7/3(VelZ) -> Terminator2/1  "GyrZ"
  Subsystem7/1(VelX) -> Square/1  "GyrX"
  Subsystem7/2(VelY) -> Square1/1  "GyrY"
  Square/1 -> Sum/1
  Square1/1 -> Sum/2
  Sum/1 -> Sqrt/1
  Sqrt/1 -> Vel_meters_ps/1

== system Main_ekart/Ref Gen ==
  VehVel_mps : Inport
  deltaSW_rad : Inport  Port=2
  Constant2 : Constant  Value=L
  Constant4 : Constant  Value=D
  reference gen : MATLAB Function  TreatAsAtomicUnit=on
  r_ref : Outport
  wires:
  Constant2/1 -> reference gen/3(L)
  Constant4/1 -> reference gen/4(D)
  VehVel_mps/1 -> reference gen/1(u)
  deltaSW_rad/1 -> reference gen/2(deltaSW)
  reference gen/1(r_ref) -> r_ref/1  "r_ref"

== system Main_ekart/Torque Allocation (Low-Level Controller) ==
  deltaT : Inport
  Tdem : Inport  Port=2
  MATLAB Function : MATLAB Function  TreatAsAtomicUnit=on
  Saturation : Saturate  UpperLimit=25*gear_ratio  LowerLimit=-25*gear_ratio
  Saturation1 : Saturate  UpperLimit=25*gear_ratio  LowerLimit=-25*gear_ratio
  TRL : Outport
  TRR : Outport  Port=2
  wires:
  deltaT/1 -> MATLAB Function/1(deltaT)
  MATLAB Function/2(TRR) -> Saturation1/1
  MATLAB Function/1(TRL) -> Saturation/1
  Tdem/1 -> MATLAB Function/2(Tdem)
  Saturation/1 -> TRL/1
  Saturation1/1 -> TRR/1

== system Main_ekart/CAN send LEFT (Throttle)/CANbegin - WARNING, CONTAINS HARDCODED VALUES ==
  Constant : Constant  Value=0  OutDataTypeStr=boolean  SampleTime=-1
  Temporary buffer : DataStoreMemory  DataStoreName=temp_1byte  ReadBeforeWriteMsg=warning  WriteAfterWriteMsg=warning  WriteAfterReadMsg=warning  ShowAdditionalParam=off  OutDataTypeStr=uint8
  Unit Delay : UnitDelay  InitialCondition=1  SampleTime=-1  HasFrameUpgradeWarning=on
  setup : Subsystem  TreatAsAtomicUnit=on
      settings: RTWSystemCode=Nonreusable function  RTWFileNameOpts=Use subsystem name
  wires:
  Unit Delay/1 -> setup/Enable
  Constant/1 -> Unit Delay/1

== system Main_ekart/CAN send LEFT (Throttle)/CANtransmit ==
  In : Inport
  CAN_ext : Inport  Port=2
  CAN_id : Inport  Port=3
  CAN_dlc : Inport  Port=4
  CAN_data : Inport  Port=5
  Temporary buffer : DataStoreMemory  DataStoreName=temp_1byte  ReadBeforeWriteMsg=warning  WriteAfterWriteMsg=warning  WriteAfterReadMsg=warning  ShowAdditionalParam=off  OutDataTypeStr=uint8
  check TxB0 : Subsystem  TreatAsAtomicUnit=on
  load Tx data : Subsystem  TreatAsAtomicUnit=on
  send TxB0 : Subsystem  TreatAsAtomicUnit=on
  Out : Outport  VectorParamsAs1DForOutWhenUnconnected=off
  CAN_Transmitted : Outport  Port=2  VectorParamsAs1DForOutWhenUnconnected=off
  wires:
  In/1 -> load Tx data/1(In1)
  load Tx data/1(Out1) -> send TxB0/1(In1)
  send TxB0/1(Out1) -> check TxB0/1(In1)
  check TxB0/1(Out1) -> Out/1
  check TxB0/2(CANTx_Transmit) -> CAN_Transmitted/1
  CAN_ext/1 -> load Tx data/2(CAN_ext)
  CAN_id/1 -> load Tx data/3(CAN_id)
  CAN_dlc/1 -> load Tx data/4(CAN_dlc)
  CAN_data/1 -> load Tx data/5(CAN_data)

== system Main_ekart/CAN send LEFT (brake)/CANbegin - WARNING, CONTAINS HARDCODED VALUES ==
  Constant : Constant  Value=0  OutDataTypeStr=boolean  SampleTime=-1
  Temporary buffer : DataStoreMemory  DataStoreName=temp_1byte  ReadBeforeWriteMsg=warning  WriteAfterWriteMsg=warning  WriteAfterReadMsg=warning  ShowAdditionalParam=off  OutDataTypeStr=uint8
  Unit Delay : UnitDelay  InitialCondition=1  SampleTime=-1  HasFrameUpgradeWarning=on
  setup : Subsystem  TreatAsAtomicUnit=on
      settings: RTWSystemCode=Nonreusable function  RTWFileNameOpts=Use subsystem name
  wires:
  Constant/1 -> Unit Delay/1
  Unit Delay/1 -> setup/Enable

== system Main_ekart/CAN send LEFT (brake)/CANtransmit ==
  In : Inport
  CAN_ext : Inport  Port=2
  CAN_id : Inport  Port=3
  CAN_dlc : Inport  Port=4
  CAN_data : Inport  Port=5
  Temporary buffer : DataStoreMemory  DataStoreName=temp_1byte  ReadBeforeWriteMsg=warning  WriteAfterWriteMsg=warning  WriteAfterReadMsg=warning  ShowAdditionalParam=off  OutDataTypeStr=uint8
  check TxB0 : Subsystem  TreatAsAtomicUnit=on
  load Tx data : Subsystem  TreatAsAtomicUnit=on
  send TxB0 : Subsystem  TreatAsAtomicUnit=on
  Out : Outport  VectorParamsAs1DForOutWhenUnconnected=off
  CAN_Transmitted : Outport  Port=2  VectorParamsAs1DForOutWhenUnconnected=off
  wires:
  CAN_data/1 -> load Tx data/5(CAN_data)
  CAN_dlc/1 -> load Tx data/4(CAN_dlc)
  CAN_id/1 -> load Tx data/3(CAN_id)
  CAN_ext/1 -> load Tx data/2(CAN_ext)
  check TxB0/2(CANTx_Transmit) -> CAN_Transmitted/1
  check TxB0/1(Out1) -> Out/1
  send TxB0/1(Out1) -> check TxB0/1(In1)
  load Tx data/1(Out1) -> send TxB0/1(In1)
  In/1 -> load Tx data/1(In1)

== system Main_ekart/CAN send RIGHT (Brake)/CANbegin - WARNING, CONTAINS HARDCODED VALUES ==
  Constant : Constant  Value=0  OutDataTypeStr=boolean  SampleTime=-1
  Temporary buffer : DataStoreMemory  DataStoreName=temp_1byte  ReadBeforeWriteMsg=warning  WriteAfterWriteMsg=warning  WriteAfterReadMsg=warning  ShowAdditionalParam=off  OutDataTypeStr=uint8
  Unit Delay : UnitDelay  InitialCondition=1  SampleTime=-1  HasFrameUpgradeWarning=on
  setup : Subsystem  TreatAsAtomicUnit=on
      settings: RTWSystemCode=Nonreusable function  RTWFileNameOpts=Use subsystem name
  wires:
  Unit Delay/1 -> setup/Enable
  Constant/1 -> Unit Delay/1

== system Main_ekart/CAN send RIGHT (Brake)/CANtransmit ==
  In : Inport
  CAN_ext : Inport  Port=2
  CAN_id : Inport  Port=3
  CAN_dlc : Inport  Port=4
  CAN_data : Inport  Port=5
  Temporary buffer : DataStoreMemory  DataStoreName=temp_1byte  ReadBeforeWriteMsg=warning  WriteAfterWriteMsg=warning  WriteAfterReadMsg=warning  ShowAdditionalParam=off  OutDataTypeStr=uint8
  check TxB0 : Subsystem  TreatAsAtomicUnit=on
  load Tx data : Subsystem  TreatAsAtomicUnit=on
  send TxB0 : Subsystem  TreatAsAtomicUnit=on
  Out : Outport  VectorParamsAs1DForOutWhenUnconnected=off
  CAN_Transmitted : Outport  Port=2  VectorParamsAs1DForOutWhenUnconnected=off
  wires:
  In/1 -> load Tx data/1(In1)
  load Tx data/1(Out1) -> send TxB0/1(In1)
  send TxB0/1(Out1) -> check TxB0/1(In1)
  check TxB0/1(Out1) -> Out/1
  check TxB0/2(CANTx_Transmit) -> CAN_Transmitted/1
  CAN_ext/1 -> load Tx data/2(CAN_ext)
  CAN_id/1 -> load Tx data/3(CAN_id)
  CAN_dlc/1 -> load Tx data/4(CAN_dlc)
  CAN_data/1 -> load Tx data/5(CAN_data)

== system Main_ekart/CAN send RIGHT (Throttle)/CANbegin - WARNING, CONTAINS HARDCODED VALUES ==
  Constant : Constant  Value=0  OutDataTypeStr=boolean  SampleTime=-1
  Temporary buffer : DataStoreMemory  DataStoreName=temp_1byte  ReadBeforeWriteMsg=warning  WriteAfterWriteMsg=warning  WriteAfterReadMsg=warning  ShowAdditionalParam=off  OutDataTypeStr=uint8
  Unit Delay : UnitDelay  InitialCondition=1  SampleTime=-1  HasFrameUpgradeWarning=on
  setup : Subsystem  TreatAsAtomicUnit=on
      settings: RTWSystemCode=Nonreusable function  RTWFileNameOpts=Use subsystem name
  wires:
  Constant/1 -> Unit Delay/1
  Unit Delay/1 -> setup/Enable

== system Main_ekart/CAN send RIGHT (Throttle)/CANtransmit ==
  In : Inport
  CAN_ext : Inport  Port=2
  CAN_id : Inport  Port=3
  CAN_dlc : Inport  Port=4
  CAN_data : Inport  Port=5
  Temporary buffer : DataStoreMemory  DataStoreName=temp_1byte  ReadBeforeWriteMsg=warning  WriteAfterWriteMsg=warning  WriteAfterReadMsg=warning  ShowAdditionalParam=off  OutDataTypeStr=uint8
  check TxB0 : Subsystem  TreatAsAtomicUnit=on
  load Tx data : Subsystem  TreatAsAtomicUnit=on
  send TxB0 : Subsystem  TreatAsAtomicUnit=on
  Out : Outport  VectorParamsAs1DForOutWhenUnconnected=off
  CAN_Transmitted : Outport  Port=2  VectorParamsAs1DForOutWhenUnconnected=off
  wires:
  CAN_data/1 -> load Tx data/5(CAN_data)
  CAN_dlc/1 -> load Tx data/4(CAN_dlc)
  CAN_id/1 -> load Tx data/3(CAN_id)
  CAN_ext/1 -> load Tx data/2(CAN_ext)
  check TxB0/2(CANTx_Transmit) -> CAN_Transmitted/1
  check TxB0/1(Out1) -> Out/1
  send TxB0/1(Out1) -> check TxB0/1(In1)
  load Tx data/1(Out1) -> send TxB0/1(In1)
  In/1 -> load Tx data/1(In1)

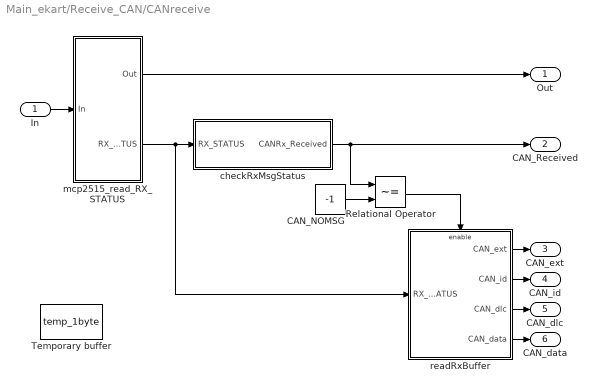
== system Main_ekart/Receive_CAN/CANreceive ==
  In : Inport
  CAN_NOMSG : Constant  Value=-1  OutDataTypeStr=int8
  Relational Operator : RelationalOperator  Operator=~=  OutDataTypeStr=boolean  RndMeth=Nearest
  Temporary buffer : DataStoreMemory  DataStoreName=temp_1byte  ReadBeforeWriteMsg=warning  WriteAfterWriteMsg=warning  WriteAfterReadMsg=warning  ShowAdditionalParam=off  OutDataTypeStr=uint8
  checkRxMsgStatus : Subsystem  TreatAsAtomicUnit=on
  mcp2515_read_RX_STATUS : Subsystem  TreatAsAtomicUnit=on
  readRxBuffer : Subsystem  TreatAsAtomicUnit=on
  Out : Outport
  CAN_Received : Outport  Port=2
  CAN_ext : Outport  Port=3
  CAN_id : Outport  Port=4
  CAN_dlc : Outport  Port=5
  CAN_data : Outport  Port=6
  wires:
  In/1 -> mcp2515_read_RX_STATUS/1(In)
  mcp2515_read_RX_STATUS/1(Out) -> Out/1
  checkRxMsgStatus/1(CANRx_Received) -> CAN_Received/1, Relational Operator/1
  mcp2515_read_RX_STATUS/2(RX_STATUS) -> readRxBuffer/1(RX_STATUS), checkRxMsgStatus/1(RX_STATUS)
  readRxBuffer/1(CAN_ext) -> CAN_ext/1
  readRxBuffer/2(CAN_id) -> CAN_id/1
  readRxBuffer/3(CAN_dlc) -> CAN_dlc/1
  readRxBuffer/4(CAN_data) -> CAN_data/1
  CAN_NOMSG/1 -> Relational Operator/2
  Relational Operator/1 -> readRxBuffer/Enable

== system Main_ekart/Receive_CAN/Subsystem ==
  CAN_Received : Inport
  CAN_EXT : Inport  Port=2
  CAN_ID : Inport  Port=3
  CAN_DLC : Inport  Port=4
  CAN_DATA : Inport  Port=5
  AND : Logic  Inputs=4  IconShape=distinctive  AllPortsSameDT=off  OutDataTypeStr=boolean
  Compare To Desired DLC : simulink/Logic and Bit Operations/Compare To Constant  relop===  const=DLC  OutDataTypeStr=boolean
  Compare To Desired DLC1 : simulink/Logic and Bit Operations/Compare To Constant  relop===  const=EXT  OutDataTypeStr=boolean
  Compare To Desired ID : simulink/Logic and Bit Operations/Compare To Constant  relop===  const=ID  OutDataTypeStr=boolean
  Memory : Memory
  Switch : Switch  Criteria=u2 > Threshold
  DATA : Outport
  wires:
  CAN_ID/1 -> Compare To Desired ID/1
  CAN_DLC/1 -> Compare To Desired DLC/1
  Compare To Desired DLC/1 -> AND/3
  Compare To Desired ID/1 -> AND/2
  CAN_Received/1 -> AND/1
  AND/1 -> Switch/2
  CAN_DATA/1 -> Switch/1
  Switch/1 -> DATA/1, Memory/1
  Memory/1 -> Switch/3
  CAN_EXT/1 -> Compare To Desired DLC1/1
  Compare To Desired DLC1/1 -> AND/4

== system Main_ekart/Receive_CAN/Subsystem1 ==
  CAN_DATA : Inport
  Byte Unpack : svdutilitieslib/Byte Unpack  dimensions={[1], [1], [1], [1], [1]}  datatypes={['uint16'], ['uint8'], ['uint8'], ['uint16'], ['uint16']}  byteAlign=1  blockPlatform=arduinoert
      settings: SourceProductBaseCode=ANDROID,ARDUINO,ML_ARDUINO,ECCORTEXA,ECCORTEXR,SC_BEAGLEBONE_BLUE,EC_FREEDOM_BOARD,EC_FRDM_K64F,INTEL_BLOCKSET,MICROBIT,NUCLEO,NVIDIA,PX4AUTOPILOTS,RASPPIIO,STMICRODIS,TIC2000,XILINX_BLOCKSET
  MATLAB Function : MATLAB Function  TreatAsAtomicUnit=on
  Terminator : Terminator
  Steering_pot_raw : Outport
  Throttle_pot_raw : Outport  Port=2
  Status_TV : Outport  Port=3
  Counter : Outport  Port=4
  wires:
  CAN_DATA/1 -> MATLAB Function/1(A)
  MATLAB Function/1(B) -> Byte Unpack/1
  Byte Unpack/1 -> Terminator/1
  Byte Unpack/2 -> Counter/1
  Byte Unpack/4 -> Throttle_pot_raw/1
  Byte Unpack/5 -> Steering_pot_raw/1
  Byte Unpack/3 -> Status_TV/1

== system Main_ekart/Receive_CAN/Subsystem2 ==
  CAN_Received : Inport
  CAN_EXT : Inport  Port=2
  CAN_ID : Inport  Port=3
  CAN_DLC : Inport  Port=4
  CAN_DATA : Inport  Port=5
  AND : Logic  Inputs=4  IconShape=distinctive  AllPortsSameDT=off  OutDataTypeStr=boolean
  Compare To Desired DLC : simulink/Logic and Bit Operations/Compare To Constant  relop===  const=DLC  OutDataTypeStr=boolean
  Compare To Desired DLC1 : simulink/Logic and Bit Operations/Compare To Constant  relop===  const=EXT  OutDataTypeStr=boolean
  Compare To Desired ID : simulink/Logic and Bit Operations/Compare To Constant  relop===  const=ID  OutDataTypeStr=boolean
  Memory : Memory
  Switch : Switch  Criteria=u2 > Threshold
  DATA : Outport
  wires:
  Compare To Desired DLC1/1 -> AND/4
  CAN_EXT/1 -> Compare To Desired DLC1/1
  Memory/1 -> Switch/3
  Switch/1 -> Memory/1, DATA/1
  CAN_DATA/1 -> Switch/1
  AND/1 -> Switch/2
  CAN_Received/1 -> AND/1
  Compare To Desired ID/1 -> AND/2
  Compare To Desired DLC/1 -> AND/3
  CAN_DLC/1 -> Compare To Desired DLC/1
  CAN_ID/1 -> Compare To Desired ID/1

== system Main_ekart/Receive_CAN/Subsystem3 ==
  Steering_pot_raw : Inport
  Constant : Constant  Value=834
  Constant1 : Constant  Value=178
  Data Type Conversion : DataTypeConversion  OutDataTypeStr=single
  MATLAB Function : MATLAB Function  TreatAsAtomicUnit=on
  Steering_angle_rad : Outport
  wires:
  MATLAB Function/1(steering_angle_rad) -> Steering_angle_rad/1
  Steering_pot_raw/1 -> Data Type Conversion/1
  Constant/1 -> MATLAB Function/1(Valpi_2)
  Constant1/1 -> MATLAB Function/3(Valnegpi_2)
  Data Type Conversion/1 -> MATLAB Function/2(steering_pot_raw)

== system Main_ekart/Receive_CAN/Subsystem4 ==
  throttle_pot_raw : Inport
  Constant : Constant  Value=233
  Constant1 : Constant  Value=640
  Data Type Conversion : DataTypeConversion  OutDataTypeStr=int16
  MATLAB Function : MATLAB Function  TreatAsAtomicUnit=on
  throttle_percent : Outport
  wires:
  Data Type Conversion/1 -> MATLAB Function/2(throttle_pot_raw)
  Constant1/1 -> MATLAB Function/3(Val0)
  Constant/1 -> MATLAB Function/1(Val100)
  throttle_pot_raw/1 -> Data Type Conversion/1
  MATLAB Function/1(throttle_percent) -> throttle_percent/1

== system Main_ekart/Receive_CAN/Subsystem5 ==
  CAN_DATA : Inport
  Byte Unpack : svdutilitieslib/Byte Unpack  dimensions={[1], [1], [1], [1]}  datatypes="{['int16'],  ['int16'], ['int16'], ['int16']}"  byteAlign=1  blockPlatform=arduinoert
      settings: SourceProductBaseCode=ANDROID,ARDUINO,ML_ARDUINO,ECCORTEXA,ECCORTEXR,SC_BEAGLEBONE_BLUE,EC_FREEDOM_BOARD,EC_FRDM_K64F,INTEL_BLOCKSET,MICROBIT,NUCLEO,NVIDIA,PX4AUTOPILOTS,RASPPIIO,STMICRODIS,TIC2000,XILINX_BLOCKSET
  Data Type Conversion : DataTypeConversion  OutDataTypeStr=double
  Data Type Conversion1 : DataTypeConversion  OutDataTypeStr=double
  Data Type Conversion2 : DataTypeConversion  OutDataTypeStr=double
  MATLAB Function : MATLAB Function  TreatAsAtomicUnit=on
  Raw2phys : Gain  Gain=2^(-9)  OutDataTypeStr=Inherit: Inherit via back propagation
  Raw2phys1 : Gain  Gain=2^(-9)  OutDataTypeStr=Inherit: Inherit via back propagation
  Raw2phys2 : Gain  Gain=2^(-9)  OutDataTypeStr=Inherit: Inherit via back propagation
  Terminator : Terminator
  GyrX : Outport
  GyrY : Outport  Port=2
  GyrZ : Outport  Port=3
  wires:
  CAN_DATA/1 -> MATLAB Function/1(A)
  MATLAB Function/1(B) -> Byte Unpack/1
  Byte Unpack/1 -> Terminator/1
  Byte Unpack/2 -> Data Type Conversion/1
  Byte Unpack/3 -> Data Type Conversion1/1
  Byte Unpack/4 -> Data Type Conversion2/1
  Raw2phys/1 -> GyrZ/1
  Raw2phys1/1 -> GyrY/1
  Raw2phys2/1 -> GyrX/1
  Data Type Conversion/1 -> Raw2phys/1
  Data Type Conversion1/1 -> Raw2phys1/1
  Data Type Conversion2/1 -> Raw2phys2/1
